simulink model "MODELO_QUIZ_2"  (R2020a)
settings: Solver=FixedStepAuto  StartTime=0.0  StopTime=15  FixedStep=0.001  RelTol=1e-3
settings Model: Creator=Alejo  LastModifiedBy=USUARIO
settings DataIOCC: ReturnWorkspaceOutputs=off
settings DebuggingCC: ArithmeticOperatorsInVariantConditions=warning
settings SFSimCC: CustomCodeUndefinedFunction=UseInterfaceOnly

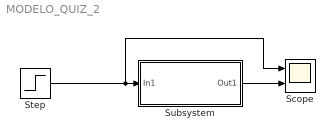
== system MODELO_QUIZ_2 ==
  Scope : Scope  NumInputPorts=2
  Step : Step  Before=1  After=0  SampleTime=0.001
  Subsystem : Subsystem
  wires:
  Step/1 -> Scope/1, Subsystem/1(In1)
  Subsystem/1(Out1) -> Scope/2

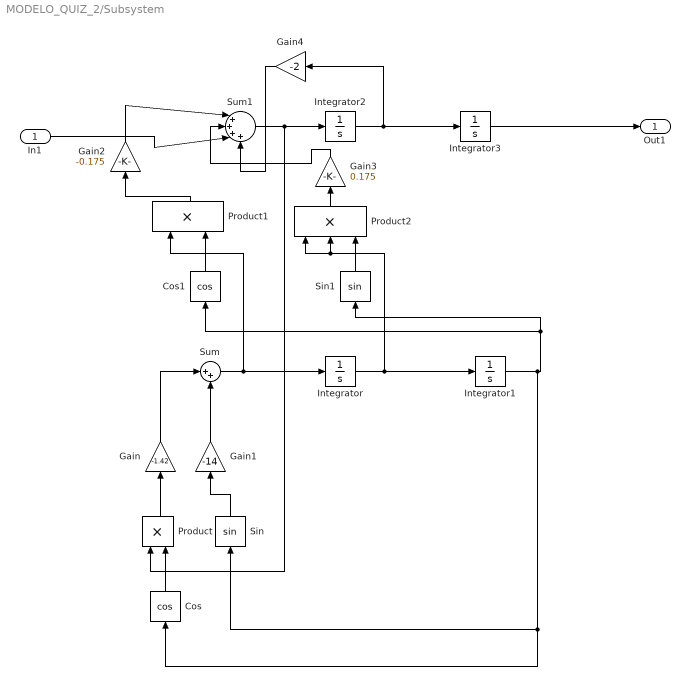
== system MODELO_QUIZ_2/Subsystem ==
  In1 : Inport
  Cos : Trigonometry  Operator=cos
  Cos1 : Trigonometry  Operator=cos
  Gain : Gain  Gain=-1.42
  Gain1 : Gain  Gain=-14
  Gain2 : Gain  Gain=-0.175
  Gain3 : Gain  Gain=0.175
  Gain4 : Gain  Gain=-2
  Integrator{,1..3} (4 alike) : Integrator
  Product : Product
  Product1 : Product
  Product2 : Product  Inputs=3
  Sin : Trigonometry
  Sin1 : Trigonometry
  Sum : Sum  Inputs=|++
  Sum1 : Sum  Inputs=|++++
  Out1 : Outport  VectorParamsAs1DForOutWhenUnconnected=off
  wires:
  Integrator/1 -> Integrator1/1, Product2/1, Product2/2
  Product2/1 -> Gain3/1
  Gain4/1 -> Sum1/4
  Cos1/1 -> Product1/2
  Gain3/1 -> Sum1/2
  Sin/1 -> Gain1/1
  Gain1/1 -> Sum/2
  Gain2/1 -> Sum1/1
  In1/1 -> Sum1/3
  Gain/1 -> Sum/1
  Sum1/1 -> Product/1, Integrator2/1
  Sin1/1 -> Product2/3
  Product/1 -> Gain/1
  Product1/1 -> Gain2/1
  Integrator2/1 -> Gain4/1, Integrator3/1
  Cos/1 -> Product/2
  Sum/1 -> Integrator/1, Product1/1
  Integrator1/1 -> Sin/1, Cos/1, Cos1/1, Sin1/1
  Integrator3/1 -> Out1/1
